simulink model "DQN_VTOL_Plant_Simulink"  (R2021a)
settings: Solver=ode1  StartTime=0.0  StopTime=Tf  FixedStep=0.01  RelTol=1e-3
InitFcn:
  | pitch0 = 0;
undefined symbols (not defined in the file or in its folder): DiscIntNeverNeededParam
libraries: rllib x1, simulink x1
settings Model: Creator=RafadanTayfa  LastModifiedBy=mluser
settings SolverCC: AlgebraicLoopSolver=TrustRegion
settings DebuggingCC: SFMachineParentedDataDiag=warning

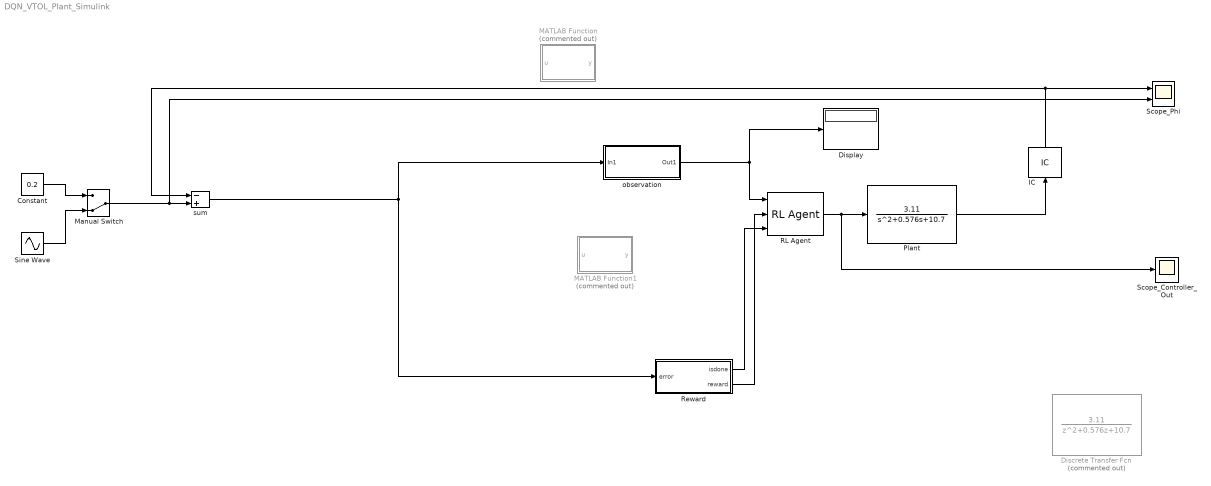
== system DQN_VTOL_Plant_Simulink ==
  Constant : Constant  Value=0.2  SampleTime=0
  Discrete Transfer Fcn : DiscreteTransferFcn  Commented=on  Numerator=[3.11]  Denominator=[1 0.576 10.7]
  Display : Display
  IC : InitialCondition  Value=pitch0
  MATLAB Function : MATLAB Function  Commented=on  TreatAsAtomicUnit=on
  MATLAB Function1 : MATLAB Function  Commented=on  TreatAsAtomicUnit=on
  Manual Switch : ManualSwitch  CurrentSetting=0
  Plant : TransferFcn  Numerator=[3.11]  Denominator=[1 0.576 10.7]
  RL Agent : rllib/RL Agent  Agent=saved_agent  ExternalActionAsInput=off  ProvideCumRwd=off  TreatAsDirectFeedthrough=on
  Reward : Subsystem
  Scope_Controller_Out : Scope
  Scope_Phi : Scope  NumInputPorts=2
  Sine Wave : Sin  Amplitude=0.2  Frequency=pi  SampleTime=0
  observation : Subsystem
  sum : Sum  Inputs=-+
  wires:
  IC/1 -> sum/1, Scope_Phi/1
  RL Agent/1 -> Plant/1, Scope_Controller_Out/1
  Manual Switch/1 -> Scope_Phi/2, sum/2
  Reward/1(isdone) -> RL Agent/3
  Plant/1 -> IC/1
  Reward/2(reward) -> RL Agent/2
  Constant/1 -> Manual Switch/1
  Sine Wave/1 -> Manual Switch/2
  sum/1 -> observation/1(In1), Reward/1(error)
  observation/1(Out1) -> Display/1, RL Agent/1

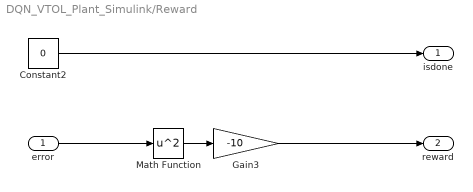
== system DQN_VTOL_Plant_Simulink/Reward ==
  error : Inport
  Constant2 : Constant  Value=0
  Gain3 : Gain  Gain=-10
  Math Function : Math  Operator=square  SignedPower=on  SaturateOnIntegerOverflow=on
  isdone : Outport  VectorParamsAs1DForOutWhenUnconnected=off
  reward : Outport  Port=2  VectorParamsAs1DForOutWhenUnconnected=off
  wires:
  Constant2/1 -> isdone/1
  error/1 -> Math Function/1
  Math Function/1 -> Gain3/1
  Gain3/1 -> reward/1

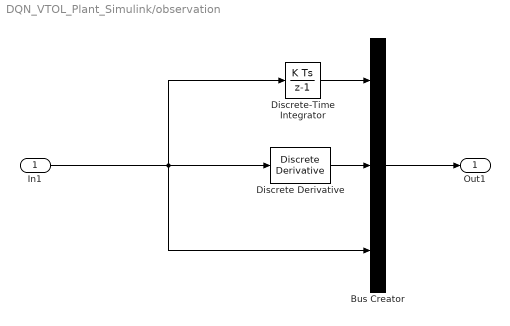
== system DQN_VTOL_Plant_Simulink/observation ==
  In1 : Inport
  Bus Creator : BusCreator  Inputs=3
  Discrete Derivative : simulink/Discrete/Discrete Derivative  gainval=1.0  ICPrevScaledInput=0.0  OutMin=[]  OutMax=[]  OutDataType=fixdt(1, 16)  OutScaling=2^-10  DoSatur=off
  Discrete-Time Integrator : DiscreteIntegrator  SampleTime=-1  ICPrevOutput=DiscIntNeverNeededParam  ICPrevScaledInput=DiscIntNeverNeededParam
  Out1 : Outport
  wires:
  In1/1 -> Bus Creator/3, Discrete Derivative/1, Discrete-Time Integrator/1
  Discrete-Time Integrator/1 -> Bus Creator/1
  Discrete Derivative/1 -> Bus Creator/2
  Bus Creator/1 -> Out1/1

== matlab function DQN_VTOL_Plant_Simulink/MATLAB Function ==
  data: u input; y output
function y= fcn(u)
    u = real(str2double(sprintf('%.4f',u)));
    if rem(u,0.001)>=5.000e-04
        u = u *1000;
        u = ceil(u);
    else
        u = u *1000;
        u = floor(u);
    end
     u = u/1000;
     y = u
end

== matlab function DQN_VTOL_Plant_Simulink/MATLAB Function1 ==
  data: u input; y output
function y= fcn(u)
    u = real(str2double(sprintf('%.4f',u)));
    y = int64(u*1000);
end
